simulink model "DBX_model_all"  (R2015a)
settings: Solver=ode2  SolverMode=SingleTasking  StartTime=0.0  StopTime=10  FixedStep=T_sim  RelTol=1e-3
undefined symbols (not defined in the file): A_M, Alpha_unique_rad, as, B_span, Beta_unique_rad, C_D_q, C_l, C_l_delta_a_Asim, C_l_delta_rv_Asim, C_l_p, C_l_r, C_Lift_q, C_m, C_m_q, C_n, C_n_delta_a_Asim, C_n_delta_rv_Asim, C_n_p, C_n_r, C_X, C_Y, C_Y_delta_rv_Asim, C_Y_p, C_Y_r, C_Z, CG, CMA, DBX_aero, DBX_aero_param, delta_elev_unique_rad, DOWN_0, EAST_0, F, g, h_1, h_2, h_3, I_BAC, Initial_Omegas, Initial_Torques, Ion, L_M, Lithium, m, MIL, NORTH_0, P_0, Q_0, R_0, Rotation_sign, Servo_calib, T_sim, U_0, V_0, W_0
libraries: simulink x19, DBX_model x14, aerolibwind2 x12, aerolibasang x9, aerolibadyn x4, aerolibatmos2 x2, powerlib x2, aerolibtransform2 x1, electricdrivelib x1
(part 2 of 3)

== system DBX_model_all/Aeromodel/Aero model V2 parametric/Wind Model ==
  note: Wind Models
  Alt (m) : Inport
  DCM : Inport  Port=2
  V_e (m/s) : Inport  Port=3
  Bias : Bias  Bias=eps
  Bias1 : Bias  Bias=eps
  Dot Product : DotProduct  SaturateOnIntegerOverflow=on  OutDataTypeStr=Inherit: Inherit via internal rule
  Dryden Wind Turbulence Model (Continuous (+q +r)) : aerolibwind2/Dryden Wind Turbulence Model  (Continuous (+q -r))  units=Metric (MKS)  spec=MIL-F-8785C  model=Continuous Von Karman (+q -r)  W20=0  Wdeg=90  TurbProb=2x10^-1  L_high=533.4  Wingspan=B_span  ts=0.2  Seed=[23341 23342 23343 23344]  T_on=on
  Horizontal Wind Model : aerolibwind2/Horizontal Wind Model  units=Metric (MKS)  Vw_source=Internal  Vwind=0  W_source=Internal  Wdeg=-60
  Sum : Sum  Inputs=+++  SaturateOnIntegerOverflow=on  InputSameDT=on  OutDataTypeStr=Inherit: Same as first input
  V : Math  Operator=sqrt  SaturateOnIntegerOverflow=on
  Wind Shear Model : aerolibwind2/Wind Shear Model  units=Metric (MKS)  phase=Category C - Terminal Flight Phase  W_20=0  Wdeg=0
  V_wind : Outport
  omega_wind : Outport  Port=2
  wires:
  Wind Shear Model/1 -> Sum/1
  Horizontal Wind Model/1 -> Sum/2
  Alt (m)/1 -> Dryden Wind Turbulence Model (Continuous (+q +r))/1, Wind Shear Model/1
  DCM/1 -> Horizontal Wind Model/1, Dryden Wind Turbulence Model (Continuous (+q +r))/3, Wind Shear Model/2
  Sum/1 -> Bias1/1
  Dryden Wind Turbulence Model (Continuous (+q +r))/2 -> omega_wind/1
  Dot Product/1 -> V/1
  V_e (m/s)/1 -> Dot Product/2, Dot Product/1
  Dryden Wind Turbulence Model (Continuous (+q +r))/1 -> Sum/3
  V/1 -> Bias/1
  Bias/1 -> Dryden Wind Turbulence Model (Continuous (+q +r))/2
  Bias1/1 -> V_wind/1

== system DBX_model_all/Aeromodel/Aero model aerosonde/Aerodynamics ==
  note: Aerodynamic Model
  note: Aerodynamic Coefficients
  note: Aerodynamic Parameters
  note: Outputs
  note: Inputs
  AeroCon : Inport  PortDimensions=[4 1]
  VelB : Inport  Port=2  PortDimensions=[3 1]
  Rates : Inport  Port=3  PortDimensions=[3 1]
  VelBdot : Inport  Port=4
  WindB : Inport  Port=5  PortDimensions=[3 1]
  WindRates : Inport  Port=6  PortDimensions=[3 1]
  rho : Inport  Port=7  PortDimensions=1
  "a " : Inport  Port=8  PortDimensions=1
  Force Coefficients : Subsystem
  Moment Coefficients : Subsystem
  Mux : Mux  Inputs=2
  Sum : Sum  Inputs=|+-  SaturateOnIntegerOverflow=on  InputSameDT=on  OutDataTypeStr=Inherit: Same as first input
  Wind-axes Velocities : Subsystem
  AeroCoeff_ba : Outport
  VelW : Outport  Port=2
  qbar (pdyn) : Outport  Port=3
  VBetaAlpha : Outport  Port=4
  wires:
  VelBdot/1 -> Wind-axes Velocities/5(VelBdot)
  Wind-axes Velocities/4(alphadot) -> Force Coefficients/3(AlphaDot), Moment Coefficients/3(AlphaDot)
  WindB/1 -> Wind-axes Velocities/2(WindB)
  Mux/1 -> AeroCoeff_ba/1
  Moment Coefficients/1("[-Cl, Cm, -Cn]") -> Mux/2
  Force Coefficients/1("[-CD, CY, -CL]") -> Mux/1
  rho/1 -> Wind-axes Velocities/4(rho)
  VelB/1 -> Wind-axes Velocities/1(VelB)
  "a "/1 -> Wind-axes Velocities/3(a)  "speed of sound"
  AeroCon/1 -> Moment Coefficients/2(Control), Force Coefficients/2(Control)
  Wind-axes Velocities/2(Mach) -> Moment Coefficients/5(Mach), Force Coefficients/5(Mach)
  Wind-axes Velocities/3(qbar (pdyn)) -> qbar (pdyn)/1
  Rates/1 -> Sum/1
  WindRates/1 -> Sum/2
  Sum/1 -> Moment Coefficients/4(AngularRates), Force Coefficients/4(AngularRates)  "pqr"
  Wind-axes Velocities/1(VBetaAlpha) -> VBetaAlpha/1, Moment Coefficients/1(VBetaAlpha), VelW/1, Force Coefficients/1(VBetaAlpha)

== system DBX_model_all/Aeromodel/Aero model aerosonde/Deflex mixer ==
  note: Control inputs:
      |
      |
      | 7. Rudervator Left (rad)
      | 8. Rudervator Right (rad)
      | 9. Aileron Left (rad)
      | 10. Aielron Right (rad)
  Sups_control : Inport
  Add : Sum  Inputs=|+-
  Add1 : Sum  Inputs=|++
  Add2 : Sum  Inputs=|+-
  Demux : Demux
  Gain : Gain  Gain=1/2
  Gain1 : Gain  Gain=1/2
  Gain2 : Gain  Gain=1/2
  delta_ail_Asim : Outport
  delta_rv_sim : Outport  Port=2
  delta_rv_Asim : Outport  Port=3
  wires:
  Sups_control/1 -> Demux/1
  Demux/3 -> Add/1
  Demux/4 -> Add/2
  Add/1 -> Gain/1
  Gain/1 -> delta_ail_Asim/1
  Demux/1 -> Add2/1, Add1/1
  Demux/2 -> Add2/2, Add1/2
  Add2/1 -> Gain1/1
  Add1/1 -> Gain2/1
  Gain2/1 -> delta_rv_sim/1
  Gain1/1 -> delta_rv_Asim/1

== system DBX_model_all/Aeromodel/Aero model aerosonde/Wind Model ==
  note: Wind Models
  Alt (m) : Inport
  DCM : Inport  Port=2
  V_e (m/s) : Inport  Port=3
  Dot Product : DotProduct  SaturateOnIntegerOverflow=on  OutDataTypeStr=Inherit: Inherit via internal rule
  Dryden Wind Turbulence Model (Continuous (+q +r)) : aerolibwind2/Dryden Wind Turbulence Model  (Continuous (+q -r))  units=Metric (MKS)  spec=MIL-F-8785C  model=Continuous Von Karman (+q -r)  W20=0  Wdeg=90  TurbProb=2x10^-1  L_high=533.4  Wingspan=B_span  ts=0.02  Seed=[23341 23342 23343 23344]  T_on=on
  Horizontal Wind Model : aerolibwind2/Horizontal Wind Model  units=Metric (MKS)  Vw_source=Internal  Vwind=0  W_source=Internal  Wdeg=-60
  Sum : Sum  Inputs=+++  SaturateOnIntegerOverflow=on  InputSameDT=on  OutDataTypeStr=Inherit: Same as first input
  V : Math  Operator=sqrt  SaturateOnIntegerOverflow=on
  Wind Shear Model : aerolibwind2/Wind Shear Model  units=Metric (MKS)  phase=Category C - Terminal Flight Phase  W_20=0  Wdeg=0
  V_wind : Outport
  omega_wind : Outport  Port=2
  wires:
  V/1 -> Dryden Wind Turbulence Model (Continuous (+q +r))/2
  Dryden Wind Turbulence Model (Continuous (+q +r))/1 -> Sum/3
  V_e (m/s)/1 -> Dot Product/2, Dot Product/1
  Dot Product/1 -> V/1
  Dryden Wind Turbulence Model (Continuous (+q +r))/2 -> omega_wind/1
  Sum/1 -> V_wind/1
  DCM/1 -> Horizontal Wind Model/1, Dryden Wind Turbulence Model (Continuous (+q +r))/3, Wind Shear Model/2
  Alt (m)/1 -> Dryden Wind Turbulence Model (Continuous (+q +r))/1, Wind Shear Model/1
  Horizontal Wind Model/1 -> Sum/2
  Wind Shear Model/1 -> Sum/1

== system DBX_model_all/Aeromodel/Aero model V1/Aerodynamics/Deflex mixer ==
  note: Control inputs:
      |
      |
      | 7. Rudervator Left (rad)
      | 8. Rudervator Right (rad)
      | 9. Aileron Left (rad)
      | 10. Aielron Right (rad)
  Sups_control : Inport
  Add : Sum  Inputs=|+-
  Add1 : Sum  Inputs=|++
  Add2 : Sum  Inputs=|+-
  Demux : Demux
  Gain : Gain  Gain=1/2
  Gain1 : Gain  Gain=1/2
  Gain2 : Gain  Gain=1/2
  delta_ail_Asim : Outport
  delta_rv_sim : Outport  Port=2
  delta_rv_Asim : Outport  Port=3
  wires:
  Sups_control/1 -> Demux/1
  Demux/3 -> Add/1
  Demux/4 -> Add/2
  Add/1 -> Gain/1
  Gain/1 -> delta_ail_Asim/1
  Demux/1 -> Add2/1, Add1/1
  Demux/2 -> Add2/2, Add1/2
  Add2/1 -> Gain1/1
  Add1/1 -> Gain2/1
  Gain2/1 -> delta_rv_sim/1
  Gain1/1 -> delta_rv_Asim/1

== system DBX_model_all/Aeromodel/Aero model V1/Aerodynamics/Force Coefficients ==
  note: Con Cariño para Luis :P
  note: Deflexiones efectivas:
      |
      | delta_ail_Asim
      | delta_rv_sim
      | delta_rv_Asim
  alpha : Inport
  beta : Inport  Port=2
  body_rates_adim : Inport  Port=3
  defl_control : Inport  Port=4
  C_X_T : Subsystem
  C_Y_T : Subsystem
  C_Z_T : Subsystem
  Mux : Mux  Inputs=3
  "[C_X_T, C_Y_T, C_Z_T]" : Outport
  wires:
  alpha/1 -> C_Z_T/1(alpha), C_Y_T/1(alpha), C_X_T/1(alpha)
  beta/1 -> C_Z_T/2(beta), C_Y_T/2(beta), C_X_T/2(beta)
  body_rates_adim/1 -> C_Z_T/3(body_rates_adim), C_Y_T/3(body_rates_adim), C_X_T/3(body_rates_adim)
  defl_control/1 -> C_Z_T/4(defl_control), C_Y_T/4(defl_control), C_X_T/4(defl_control)
  C_Y_T/1(C_Y_T) -> Mux/2
  Mux/1 -> "[C_X_T, C_Y_T, C_Z_T]"/1
  C_X_T/1(C_X_T) -> Mux/1
  C_Z_T/1(C_Z_T) -> Mux/3

== system DBX_model_all/Aeromodel/Aero model V1/Aerodynamics/Moment Coefficients ==
  note: Con Cariño para Luis :P
  note: Deflexiones efectivas:
      |
      | delta_ail_Asim
      | delta_rv_sim
      | delta_rv_Asim
  alpha : Inport
  beta : Inport  Port=2
  body_rates_adim : Inport  Port=3  PortDimensions=[3 1]
  defl_control : Inport  Port=4
  C_l_T : Subsystem
  C_m_T : Subsystem
  C_n_T : Subsystem
  Mux : Mux  Inputs=3
  "[C_l_T, C_m_T, C_n_T]" : Outport
  wires:
  alpha/1 -> C_n_T/1(alpha), C_m_T/1(alpha), C_l_T/1(alpha)
  beta/1 -> C_n_T/2(beta), C_m_T/2(beta), C_l_T/2(beta)
  body_rates_adim/1 -> C_n_T/3(body_rates_adim), C_m_T/3(body_rates_adim), C_l_T/3(body_rates_adim)
  defl_control/1 -> C_n_T/4(defl_control), C_m_T/4(defl_control), C_l_T/4(defl_control)
  Mux/1 -> "[C_l_T, C_m_T, C_n_T]"/1
  C_l_T/1(C_l_T) -> Mux/1
  C_m_T/1(C_m_T) -> Mux/2
  C_n_T/1(C_n_T) -> Mux/3

== system DBX_model_all/Aeromodel/Aero model V1/Aerodynamics/Wind-axes Velocities ==
  Vb : Inport
  V_wind_b : Inport  Port=2
  a : Inport  Port=3
  rho : Inport  Port=4
  Vb_dot : Inport  Port=5
  Calculate alphadot : Subsystem
  Derivative : Derivative  CoefficientInTFapproximation=500
  Dynamic Pressure : aerolibasang/Dynamic Pressure
  "Incidence, Sideslip, & Airspeed" : aerolibasang/Incidence, Sideslip, & Airspeed
  Sum1 : Sum  Inputs=|+-  SaturateOnIntegerOverflow=on  InputSameDT=on  OutDataTypeStr=Inherit: Same as first input
  Sum2 : Sum  Inputs=-+|  SaturateOnIntegerOverflow=on  InputSameDT=on  OutDataTypeStr=Inherit: Same as first input
  Terminator : Terminator
  qbar (pdyn) : Outport
  alphadot : Outport  Port=2
  alpha : Outport  Port=3
  beta : Outport  Port=4
  TAS : Outport  Port=5
  wires:
  Derivative/1 -> Sum2/1
  Sum2/1 -> Calculate alphadot/1("[Udot Vdot Wdot]")
  Vb_dot/1 -> Sum2/2
  Calculate alphadot/1(alphadot) -> alphadot/1
  Dynamic Pressure/1 -> qbar (pdyn)/1
  rho/1 -> Dynamic Pressure/2
  V_wind_b/1 -> Derivative/1, Sum1/2
  Vb/1 -> Sum1/1
  Sum1/1 -> Calculate alphadot/2("[U V W]"), Dynamic Pressure/1, "Incidence, Sideslip, & Airspeed"/1
  "Incidence, Sideslip, & Airspeed"/3 -> TAS/1
  "Incidence, Sideslip, & Airspeed"/2 -> beta/1
  "Incidence, Sideslip, & Airspeed"/1 -> alpha/1
  a/1 -> Terminator/1

== system DBX_model_all/Aeromodel/Aero model V2/Aerodynamics/Deflex mixer ==
  note: Control inputs:
      |
      |
      | 7. Rudervator Left (rad)
      | 8. Rudervator Right (rad)
      | 9. Aileron Left (rad)
      | 10. Aielron Right (rad)
  Sups_control : Inport
  Add : Sum  Inputs=|+-
  Add1 : Sum  Inputs=|++
  Add2 : Sum  Inputs=|+-
  Demux : Demux
  Gain : Gain  Gain=1/2
  Gain1 : Gain  Gain=1/2
  Gain2 : Gain  Gain=1/2
  delta_ail_Asim : Outport
  delta_rv_sim : Outport  Port=2
  delta_rv_Asim : Outport  Port=3
  wires:
  Gain1/1 -> delta_rv_Asim/1
  Gain2/1 -> delta_rv_sim/1
  Add1/1 -> Gain2/1
  Add2/1 -> Gain1/1
  Demux/2 -> Add1/2, Add2/2
  Demux/1 -> Add1/1, Add2/1
  Gain/1 -> delta_ail_Asim/1
  Add/1 -> Gain/1
  Demux/4 -> Add/2
  Demux/3 -> Add/1
  Sups_control/1 -> Demux/1

== system DBX_model_all/Aeromodel/Aero model V2/Aerodynamics/Force Coefficients ==
  note: Con Cariño para Luis :P
  note: Deflexiones del modelo Aero:
      |
      | delta_ail
      | delta_elev
      | delta_rudder
  alpha : Inport
  beta : Inport  Port=2
  body_rates_adim : Inport  Port=3
  defl_control : Inport  Port=4
  C_X_T : Subsystem
  C_Y_T : Subsystem
  C_Z_T : Subsystem
  Mux : Mux  Inputs=3
  "[C_X_T, C_Y_T, C_Z_T]" : Outport
  wires:
  C_Z_T/1(C_Z_T) -> Mux/3
  C_X_T/1(C_X_T) -> Mux/1
  Mux/1 -> "[C_X_T, C_Y_T, C_Z_T]"/1
  C_Y_T/1(C_Y_T) -> Mux/2
  defl_control/1 -> C_X_T/4(defl_control), C_Z_T/4(defl_control), C_Y_T/4(defl_control)
  body_rates_adim/1 -> C_X_T/3(body_rates_adim), C_Z_T/3(body_rates_adim), C_Y_T/3(body_rates_adim)
  beta/1 -> C_X_T/2(beta), C_Z_T/2(beta), C_Y_T/2(beta)
  alpha/1 -> C_X_T/1(alpha), C_Z_T/1(alpha), C_Y_T/1(alpha)

== system DBX_model_all/Aeromodel/Aero model V2/Aerodynamics/Moment Coefficients ==
  note: Con Cariño para Luis :P
  note: Deflexiones del modelo Aero:
      |
      | delta_ail
      | delta_elev
      | delta_rudder
  alpha : Inport
  beta : Inport  Port=2
  body_rates_adim : Inport  Port=3  PortDimensions=[3 1]
  defl_control : Inport  Port=4
  C_l_T : Subsystem
  C_m_T : Subsystem
  C_n_T : Subsystem
  Mux : Mux  Inputs=3
  "[C_l_T, C_m_T, C_n_T]" : Outport
  wires:
  C_n_T/1(C_n_T) -> Mux/3
  C_m_T/1(C_m_T) -> Mux/2
  C_l_T/1(C_l_T) -> Mux/1
  Mux/1 -> "[C_l_T, C_m_T, C_n_T]"/1
  defl_control/1 -> C_l_T/4(defl_control), C_n_T/4(defl_control), C_m_T/4(defl_control)
  body_rates_adim/1 -> C_l_T/3(body_rates_adim), C_n_T/3(body_rates_adim), C_m_T/3(body_rates_adim)
  beta/1 -> C_l_T/2(beta), C_n_T/2(beta), C_m_T/2(beta)
  alpha/1 -> C_l_T/1(alpha), C_n_T/1(alpha), C_m_T/1(alpha)

== system DBX_model_all/Aeromodel/Aero model V2/Aerodynamics/Wind-axes Velocities ==
  Vb : Inport
  V_wind_b : Inport  Port=2
  a : Inport  Port=3
  rho : Inport  Port=4
  Vb_dot : Inport  Port=5
  Calculate alphadot : Subsystem
  Derivative : Derivative  CoefficientInTFapproximation=500
  Dynamic Pressure : aerolibasang/Dynamic Pressure
  "Incidence, Sideslip, & Airspeed" : aerolibasang/Incidence, Sideslip, & Airspeed
  Sum1 : Sum  Inputs=|+-  SaturateOnIntegerOverflow=on  InputSameDT=on  OutDataTypeStr=Inherit: Same as first input
  Sum2 : Sum  Inputs=-+|  SaturateOnIntegerOverflow=on  InputSameDT=on  OutDataTypeStr=Inherit: Same as first input
  Terminator : Terminator
  qbar (pdyn) : Outport
  alphadot : Outport  Port=2
  alpha : Outport  Port=3
  beta : Outport  Port=4
  TAS : Outport  Port=5
  wires:
  a/1 -> Terminator/1
  "Incidence, Sideslip, & Airspeed"/1 -> alpha/1
  "Incidence, Sideslip, & Airspeed"/2 -> beta/1
  "Incidence, Sideslip, & Airspeed"/3 -> TAS/1
  Sum1/1 -> "Incidence, Sideslip, & Airspeed"/1, Dynamic Pressure/1, Calculate alphadot/2("[U V W]")
  Vb/1 -> Sum1/1
  V_wind_b/1 -> Sum1/2, Derivative/1
  rho/1 -> Dynamic Pressure/2
  Dynamic Pressure/1 -> qbar (pdyn)/1
  Calculate alphadot/1(alphadot) -> alphadot/1
  Vb_dot/1 -> Sum2/2
  Sum2/1 -> Calculate alphadot/1("[Udot Vdot Wdot]")
  Derivative/1 -> Sum2/1

== system DBX_model_all/Aeromodel/Aero model V2 parametric/Aerodynamics/Deflex mixer ==
  note: Control inputs:
      |
      |
      | 7. Rudervator Left (rad)
      | 8. Rudervator Right (rad)
      | 9. Aileron Left (rad)
      | 10. Aielron Right (rad)
  Sups_control : Inport
  Add : Sum  Inputs=|+-
  Add1 : Sum  Inputs=|++
  Add2 : Sum  Inputs=|+-
  Demux : Demux
  Gain : Gain  Gain=1/2
  Gain1 : Gain  Gain=1/2
  Gain2 : Gain  Gain=1/2
  delta_ail_Asim : Outport
  delta_rv_sim : Outport  Port=2
  delta_rv_Asim : Outport  Port=3
  wires:
  Gain1/1 -> delta_rv_Asim/1
  Gain2/1 -> delta_rv_sim/1
  Add1/1 -> Gain2/1
  Add2/1 -> Gain1/1
  Demux/2 -> Add1/2, Add2/2
  Demux/1 -> Add1/1, Add2/1
  Gain/1 -> delta_ail_Asim/1
  Add/1 -> Gain/1
  Demux/4 -> Add/2
  Demux/3 -> Add/1
  Sups_control/1 -> Demux/1

== system DBX_model_all/Aeromodel/Aero model V2 parametric/Aerodynamics/Force Coefficients ==
  note: Con Cariño para Luis :P
  note: Deflexiones del modelo Aero:
      |
      | delta_ail
      | delta_elev
      | delta_rudder
  alpha : Inport
  beta : Inport  Port=2
  body_rates_adim : Inport  Port=3
  defl_control : Inport  Port=4
  C_X_T : Subsystem
  C_Y_T : Subsystem
  C_Z_T : Subsystem
  Mux : Mux  Inputs=3
  "[C_X_T, C_Y_T, C_Z_T]" : Outport
  wires:
  C_Z_T/1(C_Z_T) -> Mux/3
  C_X_T/1(C_X_T) -> Mux/1
  Mux/1 -> "[C_X_T, C_Y_T, C_Z_T]"/1
  C_Y_T/1(C_Y_T) -> Mux/2
  defl_control/1 -> C_X_T/4(defl_control), C_Z_T/4(defl_control), C_Y_T/4(defl_control)
  body_rates_adim/1 -> C_X_T/3(body_rates_adim), C_Z_T/3(body_rates_adim), C_Y_T/3(body_rates_adim)
  beta/1 -> C_X_T/2(beta), C_Z_T/2(beta), C_Y_T/2(beta)
  alpha/1 -> C_X_T/1(alpha), C_Z_T/1(alpha), C_Y_T/1(alpha)

== system DBX_model_all/Aeromodel/Aero model V2 parametric/Aerodynamics/Moment Coefficients ==
  note: Con Cariño para Luis :P
  note: Deflexiones del modelo Aero:
      |
      | delta_ail
      | delta_elev
      | delta_rudder
  alpha : Inport
  beta : Inport  Port=2
  body_rates_adim : Inport  Port=3  PortDimensions=[3 1]
  defl_control : Inport  Port=4
  C_l_T : Subsystem
  C_m_T : Subsystem
  C_n_T : Subsystem
  Mux : Mux  Inputs=3
  "[C_l_T, C_m_T, C_n_T]" : Outport
  wires:
  C_n_T/1(C_n_T) -> Mux/3
  C_m_T/1(C_m_T) -> Mux/2
  C_l_T/1(C_l_T) -> Mux/1
  Mux/1 -> "[C_l_T, C_m_T, C_n_T]"/1
  defl_control/1 -> C_l_T/4(defl_control), C_n_T/4(defl_control), C_m_T/4(defl_control)
  body_rates_adim/1 -> C_l_T/3(body_rates_adim), C_n_T/3(body_rates_adim), C_m_T/3(body_rates_adim)
  beta/1 -> C_l_T/2(beta), C_n_T/2(beta), C_m_T/2(beta)
  alpha/1 -> C_l_T/1(alpha), C_n_T/1(alpha), C_m_T/1(alpha)

== system DBX_model_all/Aeromodel/Aero model V2 parametric/Aerodynamics/Wind-axes Velocities ==
  Vb : Inport
  V_wind_b : Inport  Port=2
  a : Inport  Port=3
  rho : Inport  Port=4
  Vb_dot : Inport  Port=5
  Calculate alphadot : Subsystem
  Derivative : Derivative  CoefficientInTFapproximation=500
  Dynamic Pressure : aerolibasang/Dynamic Pressure
  "Incidence, Sideslip, & Airspeed" : aerolibasang/Incidence, Sideslip, & Airspeed
  Sum1 : Sum  Inputs=|+-  SaturateOnIntegerOverflow=on  InputSameDT=on  OutDataTypeStr=Inherit: Same as first input
  Sum2 : Sum  Inputs=-+|  SaturateOnIntegerOverflow=on  InputSameDT=on  OutDataTypeStr=Inherit: Same as first input
  Terminator : Terminator
  qbar (pdyn) : Outport
  alphadot : Outport  Port=2
  alpha : Outport  Port=3
  beta : Outport  Port=4
  TAS : Outport  Port=5
  wires:
  a/1 -> Terminator/1
  "Incidence, Sideslip, & Airspeed"/1 -> alpha/1
  "Incidence, Sideslip, & Airspeed"/2 -> beta/1
  "Incidence, Sideslip, & Airspeed"/3 -> TAS/1
  Sum1/1 -> "Incidence, Sideslip, & Airspeed"/1, Dynamic Pressure/1, Calculate alphadot/2("[U V W]")
  Vb/1 -> Sum1/1
  V_wind_b/1 -> Sum1/2, Derivative/1
  rho/1 -> Dynamic Pressure/2
  Dynamic Pressure/1 -> qbar (pdyn)/1
  Calculate alphadot/1(alphadot) -> alphadot/1
  Vb_dot/1 -> Sum2/2
  Sum2/1 -> Calculate alphadot/1("[Udot Vdot Wdot]")
  Derivative/1 -> Sum2/1

== system DBX_model_all/Aeromodel/Aero model aerosonde/Aerodynamics/Force Coefficients ==
  note: Force coefficients
  VBetaAlpha : Inport  PortDimensions=[3 1]
  Control : Inport  Port=2  PortDimensions=[4 1]
  AlphaDot : Inport  Port=3
  AngularRates : Inport  Port=4  PortDimensions=[3 1]
  Mach : Inport  Port=5  PortDimensions=1
  2c : Gain  Gain=2  SaturateOnIntegerOverflow=on  OutDataTypeStr=Inherit: Same as input  ParamDataTypeStr=Inherit: Same as input
  ChSign : Gain  Gain=-1  SaturateOnIntegerOverflow=on  OutDataTypeStr=Inherit: Same as input  ParamDataTypeStr=Inherit: Same as input
  ChSign1 : Gain  Gain=-1  SaturateOnIntegerOverflow=on  OutDataTypeStr=Inherit: Same as input  ParamDataTypeStr=Inherit: Same as input
  DCM' : Math  Operator=transpose  SaturateOnIntegerOverflow=on
  Demux2 : Demux  Outputs=3
  Direction Cosine Matrix Body to Wind : aerolibtransform2/Direction Cosine Matrix Body to Wind
  Drag Coefficients : Subsystem
  Lift Coefficients : Subsystem
  Mux : Mux  Inputs=3
  Mux1 : Mux  Inputs=2
  Side Force Coefficients : Subsystem
  transform to body axes : Product  Inputs=**  Multiplication=Matrix(*)  SaturateOnIntegerOverflow=on  InputSameDT=on  OutDataTypeStr=Inherit: Same as first input
  "[-CD, CY, -CL]" : Outport
  wires:
  Mux1/1 -> Direction Cosine Matrix Body to Wind/1
  DCM'/1 -> transform to body axes/1
  Mux/1 -> transform to body axes/2
  Direction Cosine Matrix Body to Wind/1 -> DCM'/1
  transform to body axes/1 -> "[-CD, CY, -CL]"/1
  Demux2/2 -> Mux1/2, Side Force Coefficients/1(beta)
  Demux2/1 -> 2c/1
  VBetaAlpha/1 -> Demux2/1
  ChSign1/1 -> Mux/3
  ChSign/1 -> Mux/1
  Side Force Coefficients/1(CY) -> Mux/2
  Drag Coefficients/1(CD) -> ChSign/1
  Lift Coefficients/1(CL) -> Drag Coefficients/3(CL), ChSign1/1
  Mach/1 -> Drag Coefficients/2(Mach), Lift Coefficients/6(Mach)
  AngularRates/1 -> Side Force Coefficients/3(angular rates), Lift Coefficients/4(pqr)
  AlphaDot/1 -> Lift Coefficients/3(alphadot)
  Control/1 -> Side Force Coefficients/2(control), Lift Coefficients/2(control), Drag Coefficients/1(control)
  Demux2/3 -> Lift Coefficients/1(alpha), Mux1/1
  2c/1 -> Side Force Coefficients/4(2V_a), Lift Coefficients/5(2V_a)

== system DBX_model_all/Aeromodel/Aero model aerosonde/Aerodynamics/Moment Coefficients ==
  note: Moment coefficients
  VBetaAlpha : Inport  PortDimensions=[3 1]
  Control : Inport  Port=2  PortDimensions=[4 1]
  AlphaDot : Inport  Port=3
  AngularRates : Inport  Port=4  PortDimensions=[3 1]
  Mach : Inport  Port=5  PortDimensions=1
  2c : Gain  Gain=2  SaturateOnIntegerOverflow=on  OutDataTypeStr=Inherit: Same as input  ParamDataTypeStr=Inherit: Same as input
  Demux1 : Demux  Outputs=3
  Mux : Mux  Inputs=3
  Pitch Moment Coefficients : Subsystem
  Roll Moment Coefficients : Subsystem
  Yaw Moment Coefficients : Subsystem
  "[-Cl, Cm, -Cn]" : Outport
  wires:
  Demux1/2 -> Yaw Moment Coefficients/1(beta), Roll Moment Coefficients/1(beta)
  Demux1/3 -> Pitch Moment Coefficients/1(alpha)
  Mach/1 -> Pitch Moment Coefficients/6(Mach)
  Yaw Moment Coefficients/1(Cn) -> Mux/3
  VBetaAlpha/1 -> Demux1/1
  2c/1 -> Pitch Moment Coefficients/5(2V_a), Yaw Moment Coefficients/4(2V_a), Roll Moment Coefficients/4(2V)
  Demux1/1 -> 2c/1
  Control/1 -> Yaw Moment Coefficients/2(control), Pitch Moment Coefficients/2(control), Roll Moment Coefficients/2(control)
  AlphaDot/1 -> Pitch Moment Coefficients/3(alphadot)
  AngularRates/1 -> Roll Moment Coefficients/3(angular rates), Yaw Moment Coefficients/3(angular rates), Pitch Moment Coefficients/4(pqr)
  Mux/1 -> "[-Cl, Cm, -Cn]"/1
  Pitch Moment Coefficients/1(Cm) -> Mux/2
  Roll Moment Coefficients/1(Cl) -> Mux/1

== system DBX_model_all/Aeromodel/Aero model aerosonde/Aerodynamics/Wind-axes Velocities ==
  VelB : Inport
  WindB : Inport  Port=2
  a : Inport  Port=3
  rho : Inport  Port=4
  VelBdot : Inport  Port=5
  Calculate alphadot : Subsystem
  Derivative : Derivative
  Dynamic Pressure : aerolibasang/Dynamic Pressure
  "Incidence, Sideslip, & Airspeed" : aerolibasang/Incidence, Sideslip, & Airspeed
  Mach Number : aerolibasang/Mach Number
  Mux1 : Mux  Inputs=3
  Sum1 : Sum  Inputs=|+-  SaturateOnIntegerOverflow=on  InputSameDT=on  OutDataTypeStr=Inherit: Same as first input
  Sum2 : Sum  Inputs=-+|  SaturateOnIntegerOverflow=on  InputSameDT=on  OutDataTypeStr=Inherit: Same as first input
  VBetaAlpha : Outport
  Mach : Outport  Port=2
  qbar (pdyn) : Outport  Port=3
  alphadot : Outport  Port=4
  wires:
  Derivative/1 -> Sum2/1
  Sum2/1 -> Calculate alphadot/1("[Udot Vdot Wdot]")
  VelBdot/1 -> Sum2/2
  Calculate alphadot/1(alphadot) -> alphadot/1
  "Incidence, Sideslip, & Airspeed"/2 -> Mux1/2
  "Incidence, Sideslip, & Airspeed"/1 -> Mux1/3
  Dynamic Pressure/1 -> qbar (pdyn)/1
  rho/1 -> Dynamic Pressure/2
  a/1 -> Mach Number/2
  Mach Number/1 -> Mach/1
  WindB/1 -> Derivative/1, Sum1/2
  VelB/1 -> Sum1/1
  Mux1/1 -> VBetaAlpha/1
  "Incidence, Sideslip, & Airspeed"/3 -> Mux1/1
  Sum1/1 -> Calculate alphadot/2("[U V W]"), Dynamic Pressure/1, Mach Number/1, "Incidence, Sideslip, & Airspeed"/1

== system DBX_model_all/Aeromodel/Aero model V1/Aerodynamics/Force Coefficients/C_X_T ==
  note: Deflexiones efectivas:
      |
      | delta_ail_Asim
      | delta_rv_sim
      | delta_rv_Asim
  alpha : Inport
  beta : Inport  Port=2
  body_rates_adim : Inport  Port=3  PortDimensions=[3 1]
  defl_control : Inport  Port=4
  Add : Sum  Inputs=++|
  Add1 : Sum  Inputs=-+|
  C_D_q : Constant  Value=C_D_q
  C_Lift_q : Constant  Value=C_Lift_q
  C_X : Lookup_n-D  NumberOfTableDimensions=3  BreakpointsForDimension1=Alpha_unique_rad  BreakpointsForDimension2=Beta_unique_rad  BreakpointsForDimension3=delta_elev_unique_rad  Table=C_X  DiagnosticForOutOfRangeInput=Warning  RemoveProtectionInput=on  InternalRulePriority=Speed  RndMeth=Simplest  InputSameDT=on
  Divide : Product  Inputs=**
  Divide1 : Product  Inputs=**
  Divide2 : Product  Inputs=**
  Selector : Selector  InputPortWidth=3  Indices=2
  Selector1 : Selector  InputPortWidth=3  Indices=2
  cos : Trigonometry  Operator=cos
  sin : Trigonometry
  C_X_T : Outport
  wires:
  alpha/1 -> cos/1, sin/1, C_X/1
  beta/1 -> C_X/2
  body_rates_adim/1 -> Selector/1
  Selector/1 -> Divide/1
  C_X/1 -> Add/1
  Divide/1 -> Add/2
  Add/1 -> C_X_T/1
  defl_control/1 -> Selector1/1
  Selector1/1 -> C_X/3
  sin/1 -> Divide1/1
  C_Lift_q/1 -> Divide1/2
  cos/1 -> Divide2/1
  C_D_q/1 -> Divide2/2
  Divide1/1 -> Add1/2
  Divide2/1 -> Add1/1
  Add1/1 -> Divide/2

== system DBX_model_all/Aeromodel/Aero model V1/Aerodynamics/Force Coefficients/C_Y_T ==
  note: Deflexiones efectivas:
      |
      | delta_ail_Asim
      | delta_rv_sim
      | delta_rv_Asim
  alpha : Inport
  beta : Inport  Port=2
  body_rates_adim : Inport  Port=3  PortDimensions=[3 1]
  defl_control : Inport  Port=4
  Add : Sum  Inputs=++++
  C_Y : Lookup_n-D  BreakpointsForDimension1=Alpha_unique_rad  BreakpointsForDimension2=Beta_unique_rad  Table=C_Y  DiagnosticForOutOfRangeInput=Warning  RemoveProtectionInput=on  InternalRulePriority=Speed  RndMeth=Simplest  InputSameDT=on
  C_Y_delta_rv : Constant  Value=C_Y_delta_rv_Asim
  C_Y_p : Constant  Value=C_Y_p
  C_Y_r : Constant  Value=C_Y_r
  Divide : Product  Inputs=**
  Divide1 : Product  Inputs=**
  Divide2 : Product  Inputs=**
  Selector : Selector  InputPortWidth=3  Indices=3
  Selector1 : Selector  InputPortWidth=3
  Selector2 : Selector  InputPortWidth=3  Indices=3
  C_Y_T : Outport
  wires:
  alpha/1 -> C_Y/1
  beta/1 -> C_Y/2
  Selector/1 -> Divide/1
  C_Y_r/1 -> Divide/2
  body_rates_adim/1 -> Selector1/1, Selector/1
  Selector1/1 -> Divide1/1
  C_Y_p/1 -> Divide1/2
  defl_control/1 -> Selector2/1
  C_Y_delta_rv/1 -> Divide2/2
  Selector2/1 -> Divide2/1
  Divide2/1 -> Add/4
  Divide1/1 -> Add/3
  Divide/1 -> Add/2
  C_Y/1 -> Add/1
  Add/1 -> C_Y_T/1

== system DBX_model_all/Aeromodel/Aero model V1/Aerodynamics/Force Coefficients/C_Z_T ==
  note: Deflexiones efectivas:
      |
      | delta_ail_Asim
      | delta_rv_sim
      | delta_rv_Asim
  alpha : Inport
  beta : Inport  Port=2
  body_rates_adim : Inport  Port=3  PortDimensions=[3 1]
  defl_control : Inport  Port=4
  Add : Sum  Inputs=++|
  Add1 : Sum  Inputs=--|
  C_D_q : Constant  Value=C_D_q
  C_Lift_q : Constant  Value=C_Lift_q
  C_Z : Lookup_n-D  NumberOfTableDimensions=3  BreakpointsForDimension1=Alpha_unique_rad  BreakpointsForDimension2=Beta_unique_rad  BreakpointsForDimension3=delta_elev_unique_rad  Table=C_Z  DiagnosticForOutOfRangeInput=Warning  RemoveProtectionInput=on  InternalRulePriority=Speed  RndMeth=Simplest  InputSameDT=on
  Divide : Product  Inputs=**
  Divide1 : Product  Inputs=**
  Divide2 : Product  Inputs=**
  Selector : Selector  InputPortWidth=3  Indices=2
  Selector1 : Selector  InputPortWidth=3  Indices=2
  cos : Trigonometry  Operator=cos
  sin : Trigonometry
  C_Z_T : Outport
  wires:
  Add/1 -> C_Z_T/1
  Divide/1 -> Add/2
  C_Z/1 -> Add/1
  Selector/1 -> Divide/1
  body_rates_adim/1 -> Selector/1
  beta/1 -> C_Z/2
  alpha/1 -> cos/1, sin/1, C_Z/1
  defl_control/1 -> Selector1/1
  Selector1/1 -> C_Z/3
  cos/1 -> Divide1/1
  C_Lift_q/1 -> Divide1/2
  C_D_q/1 -> Divide2/2
  Divide1/1 -> Add1/2
  Divide2/1 -> Add1/1
  sin/1 -> Divide2/1
  Add1/1 -> Divide/2

== system DBX_model_all/Aeromodel/Aero model V1/Aerodynamics/Moment Coefficients/C_l_T ==
  note: Deflexiones efectivas:
      |
      | delta_ail_Asim
      | delta_rv_sim
      | delta_rv_Asim
  alpha : Inport
  beta : Inport  Port=2
  body_rates_adim : Inport  Port=3  PortDimensions=[3 1]
  defl_control : Inport  Port=4
  Add : Sum  Inputs=+++++
  C_l : Lookup_n-D  BreakpointsForDimension1=Alpha_unique_rad  BreakpointsForDimension2=Beta_unique_rad  Table=C_l  DiagnosticForOutOfRangeInput=Warning  RemoveProtectionInput=on  InternalRulePriority=Speed  RndMeth=Simplest  InputSameDT=on
  C_l_delta_a : Constant  Value=C_l_delta_a_Asim
  C_l_delta_rv : Constant  Value=C_l_delta_rv_Asim
  C_l_p : Constant  Value=C_l_p
  C_l_r : Constant  Value=C_l_r
  Divide{,1..3} (4 alike) : Product  Inputs=**
  Selector : Selector  InputPortWidth=3  Indices=3
  Selector1 : Selector  InputPortWidth=3  Indices=3
  Selector2 : Selector  InputPortWidth=3
  Selector3 : Selector  InputPortWidth=3
  C_l_T : Outport
  wires:
  alpha/1 -> C_l/1
  beta/1 -> C_l/2
  Add/1 -> C_l_T/1
  defl_control/1 -> Selector1/1, Selector2/1
  C_l_delta_a/1 -> Divide2/2
  Selector2/1 -> Divide2/1
  C_l_delta_rv/1 -> Divide1/2
  Selector1/1 -> Divide1/1
  C_l_r/1 -> Divide/2
  body_rates_adim/1 -> Selector3/1, Selector/1
  Selector3/1 -> Divide3/1
  C_l_p/1 -> Divide3/2
  Selector/1 -> Divide/1
  C_l/1 -> Add/1
  Divide/1 -> Add/2
  Divide3/1 -> Add/3
  Divide2/1 -> Add/4
  Divide1/1 -> Add/5

== system DBX_model_all/Aeromodel/Aero model V1/Aerodynamics/Moment Coefficients/C_m_T ==
  note: Deflexiones efectivas:
      |
      | delta_ail_Asim
      | delta_rv_sim
      | delta_rv_Asim
  alpha : Inport
  beta : Inport  Port=2
  body_rates_adim : Inport  Port=3  PortDimensions=[3 1]
  defl_control : Inport  Port=4
  Add : Sum  Inputs=++|
  C_m : Lookup_n-D  NumberOfTableDimensions=3  BreakpointsForDimension1=Alpha_unique_rad  BreakpointsForDimension2=Beta_unique_rad  BreakpointsForDimension3=delta_elev_unique_rad  Table=C_m  DiagnosticForOutOfRangeInput=Warning  RemoveProtectionInput=on  InternalRulePriority=Speed  RndMeth=Simplest  InputSameDT=on
  C_m_q : Constant  Value=C_m_q
  Divide : Product  Inputs=**
  Selector : Selector  InputPortWidth=3  Indices=2
  Selector2 : Selector  InputPortWidth=3  Indices=2
  C_m_T : Outport
  wires:
  alpha/1 -> C_m/1
  Selector/1 -> Divide/1
  C_m_q/1 -> Divide/2
  body_rates_adim/1 -> Selector/1
  defl_control/1 -> Selector2/1
  Divide/1 -> Add/2
  C_m/1 -> Add/1
  Add/1 -> C_m_T/1
  Selector2/1 -> C_m/3
  beta/1 -> C_m/2

== system DBX_model_all/Aeromodel/Aero model V1/Aerodynamics/Moment Coefficients/C_n_T ==
  note: Deflexiones efectivas:
      |
      | delta_ail_Asim
      | delta_rv_sim
      | delta_rv_Asim
  alpha : Inport
  beta : Inport  Port=2
  body_rates_adim : Inport  Port=3  PortDimensions=[3 1]
  defl_control : Inport  Port=4
  Add : Sum  Inputs=+++++
  C_n : Lookup_n-D  BreakpointsForDimension1=Alpha_unique_rad  BreakpointsForDimension2=Beta_unique_rad  Table=C_n  DiagnosticForOutOfRangeInput=Warning  RemoveProtectionInput=on  InternalRulePriority=Speed  RndMeth=Simplest  InputSameDT=on
  C_n_delta_a : Constant  Value=C_n_delta_a_Asim
  C_n_delta_rv : Constant  Value=C_n_delta_rv_Asim
  C_n_p : Constant  Value=C_n_p
  C_n_r : Constant  Value=C_n_r
  Divide{,1..3} (4 alike) : Product  Inputs=**
  Selector : Selector  InputPortWidth=3  Indices=3
  Selector1 : Selector  InputPortWidth=3  Indices=3
  Selector2 : Selector  InputPortWidth=3
  Selector3 : Selector  InputPortWidth=3
  C_n_T : Outport
  wires:
  alpha/1 -> C_n/1
  beta/1 -> C_n/2
  Add/1 -> C_n_T/1
  defl_control/1 -> Selector1/1, Selector2/1
  C_n_delta_a/1 -> Divide2/2
  Selector2/1 -> Divide2/1
  C_n_delta_rv/1 -> Divide1/2
  Selector1/1 -> Divide1/1
  C_n_r/1 -> Divide/2
  body_rates_adim/1 -> Selector3/1, Selector/1
  Selector3/1 -> Divide3/1
  C_n_p/1 -> Divide3/2
  Selector/1 -> Divide/1
  C_n/1 -> Add/1
  Divide/1 -> Add/2
  Divide3/1 -> Add/3
  Divide2/1 -> Add/4
  Divide1/1 -> Add/5

== system DBX_model_all/Aeromodel/Aero model V1/Aerodynamics/Wind-axes Velocities/Calculate alphadot ==
  note: Calculate alphadot
  note: W
  "[Udot Vdot Wdot]" : Inport
  "[U V W]" : Inport  Port=2
  Demux : Demux  Outputs=3
  Demux1 : Demux  Outputs=3
  Math Function : Math  Operator=square  SaturateOnIntegerOverflow=on
  Math Function1 : Math  Operator=square  SaturateOnIntegerOverflow=on
  Product : Product  RndMeth=Zero
  Product1 : Product  RndMeth=Zero
  Product2 : Product  Inputs=*/  RndMeth=Zero
  Sum : Sum  Inputs=-|+
  Sum1 : Sum  Inputs=+|+
  Terminator : Terminator
  Terminator1 : Terminator
  alphadot : Outport
  wires:
  Product2/1 -> alphadot/1  "alphadot"
  "[Udot Vdot Wdot]"/1 -> Demux/1
  "[U V W]"/1 -> Demux1/1
  Demux1/2 -> Terminator1/1
  Sum/1 -> Product2/1
  Product/1 -> Sum/2  "U Wdot"
  Product1/1 -> Sum/1  "W Udot"
  Sum1/1 -> Product2/2  "U^2 + W^2"
  Math Function1/1 -> Sum1/2
  Math Function/1 -> Sum1/1
  Demux1/3 -> Math Function1/1, Product1/2
  Demux1/1 -> Math Function/1, Product/2  "U"
  Demux/2 -> Terminator/1
  Demux/3 -> Product/1  "Wdot"
  Demux/1 -> Product1/1  "Udot"

== system DBX_model_all/Aeromodel/Aero model V2/Aerodynamics/Force Coefficients/C_X_T ==
  note: Deflexiones del modelo Aero:
      |
      | delta_ail
      | delta_elev
      | delta_rudder
  alpha : Inport
  beta : Inport  Port=2
  body_rates_adim : Inport  Port=3  PortDimensions=[3 1]
  defl_control : Inport  Port=4
  Abs : Abs
  Add : Sum  Inputs=+++
  Add1 : Sum  Inputs=-+|
  C_D_q : Constant  Value=DBX_aero.C_D_q
  C_Lift_q : Constant  Value=DBX_aero.C_Lift_q
  C_X : Lookup_n-D  BreakpointsForDimension1=DBX_aero.alpha_rad  BreakpointsForDimension2=DBX_aero.beta_rad  BreakpointsForDimension3=delta_elev_unique_rad  BeginIndexSearchUsingPreviousIndexResult=on  Table=DBX_aero.C_X  ExtrapMethod=Clip  DiagnosticForOutOfRangeInput=Warning  RemoveProtectionInput=on  InternalRulePriority=Speed  RndMeth=Simplest  InputSameDT=on
  C_X_delta_elev : Lookup_n-D  BreakpointsForDimension1=DBX_aero.alpha_rad  BreakpointsForDimension2=DBX_aero.delta_elev_rad  BreakpointsForDimension3=delta_elev_unique_rad  BeginIndexSearchUsingPreviousIndexResult=on  Table=DBX_aero.C_X_delta_elev  ExtrapMethod=Clip  DiagnosticForOutOfRangeInput=Warning  RemoveProtectionInput=on  InternalRulePriority=Speed  RndMeth=Simplest  InputSameDT=on
  Divide : Product  Inputs=**
  Divide1 : Product  Inputs=**
  Divide2 : Product  Inputs=**
  Selector : Selector  InputPortWidth=3  Indices=2
  Selector1 : Selector  InputPortWidth=3  Indices=2
  cos : Trigonometry  Operator=cos
  sin : Trigonometry
  C_X_T : Outport
  wires:
  Divide2/1 -> Add1/1
  Divide1/1 -> Add1/2
  C_D_q/1 -> Divide2/2
  cos/1 -> Divide2/1
  C_Lift_q/1 -> Divide1/2
  sin/1 -> Divide1/1
  defl_control/1 -> Selector1/1
  Add/1 -> C_X_T/1
  Divide/1 -> Add/3
  Selector/1 -> Divide/2
  body_rates_adim/1 -> Selector/1
  beta/1 -> Abs/1
  alpha/1 -> cos/1, C_X_delta_elev/1, sin/1, C_X/1
  Selector1/1 -> C_X_delta_elev/2
  C_X_delta_elev/1 -> Add/2
  Add1/1 -> Divide/1
  C_X/1 -> Add/1
  Abs/1 -> C_X/2

== system DBX_model_all/Aeromodel/Aero model V2/Aerodynamics/Force Coefficients/C_Y_T ==
  note: Deflexiones del modelo Aero:
      |
      | delta_ail
      | delta_elev
      | delta_rudder
  alpha : Inport
  beta : Inport  Port=2
  body_rates_adim : Inport  Port=3  PortDimensions=[3 1]
  defl_control : Inport  Port=4
  Abs : Abs
  Add : Sum  Inputs=++++
  C_Y : Lookup_n-D  BreakpointsForDimension1=DBX_aero.alpha_rad  BreakpointsForDimension2=DBX_aero.beta_rad  BreakpointsForDimension3=delta_elev_unique_rad  BeginIndexSearchUsingPreviousIndexResult=on  Table=DBX_aero.C_Y  ExtrapMethod=Clip  DiagnosticForOutOfRangeInput=Warning  RemoveProtectionInput=on  InternalRulePriority=Speed  RndMeth=Simplest  InputSameDT=on
  C_Y_delta_rudd : Constant  Value=DBX_aero.C_Y_delta_rud
  C_Y_p : Constant  Value=DBX_aero.C_Y_p
  C_Y_r : Constant  Value=DBX_aero.C_Y_r
  Divide : Product  Inputs=**
  Divide1 : Product  Inputs=**
  Divide2 : Product  Inputs=**
  Product : Product
  Selector : Selector  InputPortWidth=3  Indices=3
  Selector1 : Selector  InputPortWidth=3
  Selector2 : Selector  InputPortWidth=3  Indices=3
  Sign : Signum
  C_Y_T : Outport
  wires:
  Add/1 -> C_Y_T/1
  Divide/1 -> Add/2
  Divide1/1 -> Add/3
  Divide2/1 -> Add/4
  Selector2/1 -> Divide2/1
  C_Y_delta_rudd/1 -> Divide2/2
  defl_control/1 -> Selector2/1
  C_Y_p/1 -> Divide1/2
  Selector1/1 -> Divide1/1
  body_rates_adim/1 -> Selector/1, Selector1/1
  C_Y_r/1 -> Divide/2
  Selector/1 -> Divide/1
  beta/1 -> Sign/1, Abs/1
  alpha/1 -> C_Y/1
  Sign/1 -> Product/2
  C_Y/1 -> Product/1
  Product/1 -> Add/1
  Abs/1 -> C_Y/2

== system DBX_model_all/Aeromodel/Aero model V2/Aerodynamics/Force Coefficients/C_Z_T ==
  note: Deflexiones del modelo Aero:
      |
      | delta_ail
      | delta_elev
      | delta_rudder
  alpha : Inport
  beta : Inport  Port=2
  body_rates_adim : Inport  Port=3  PortDimensions=[3 1]
  defl_control : Inport  Port=4
  Abs : Abs
  Add : Sum  Inputs=+++
  Add2 : Sum  Inputs=--|
  C_D_q : Constant  Value=DBX_aero.C_D_q
  C_Lift_q : Constant  Value=DBX_aero.C_Lift_q
  C_Z : Lookup_n-D  BreakpointsForDimension1=DBX_aero.alpha_rad  BreakpointsForDimension2=DBX_aero.beta_rad  BreakpointsForDimension3=delta_elev_unique_rad  BeginIndexSearchUsingPreviousIndexResult=on  Table=DBX_aero.C_Z  ExtrapMethod=Clip  DiagnosticForOutOfRangeInput=Warning  RemoveProtectionInput=on  InternalRulePriority=Speed  RndMeth=Simplest  InputSameDT=on
  C_Z_delta_elev : Lookup_n-D  BreakpointsForDimension1=DBX_aero.alpha_rad  BreakpointsForDimension2=DBX_aero.delta_elev_rad  BreakpointsForDimension3=delta_elev_unique_rad  BeginIndexSearchUsingPreviousIndexResult=on  Table=DBX_aero.C_Z_delta_elev  ExtrapMethod=Clip  DiagnosticForOutOfRangeInput=Warning  RemoveProtectionInput=on  InternalRulePriority=Speed  RndMeth=Simplest  InputSameDT=on
  Divide : Product  Inputs=**
  Divide4 : Product  Inputs=**
  Divide5 : Product  Inputs=**
  Selector : Selector  InputPortWidth=3  Indices=2
  Selector1 : Selector  InputPortWidth=3  Indices=2
  cos1 : Trigonometry  Operator=cos
  sin1 : Trigonometry
  C_Z_T : Outport
  wires:
  Add2/1 -> Divide/1
  C_Z_delta_elev/1 -> Add/2
  Selector1/1 -> C_Z_delta_elev/2
  beta/1 -> Abs/1
  body_rates_adim/1 -> Selector/1
  Selector/1 -> Divide/2
  Divide/1 -> Add/3
  Add/1 -> C_Z_T/1
  defl_control/1 -> Selector1/1
  sin1/1 -> Divide5/1
  Divide5/1 -> Add2/1
  Divide4/1 -> Add2/2
  C_D_q/1 -> Divide5/2
  C_Lift_q/1 -> Divide4/2
  cos1/1 -> Divide4/1
  alpha/1 -> C_Z/1, C_Z_delta_elev/1, sin1/1, cos1/1
  C_Z/1 -> Add/1
  Abs/1 -> C_Z/2

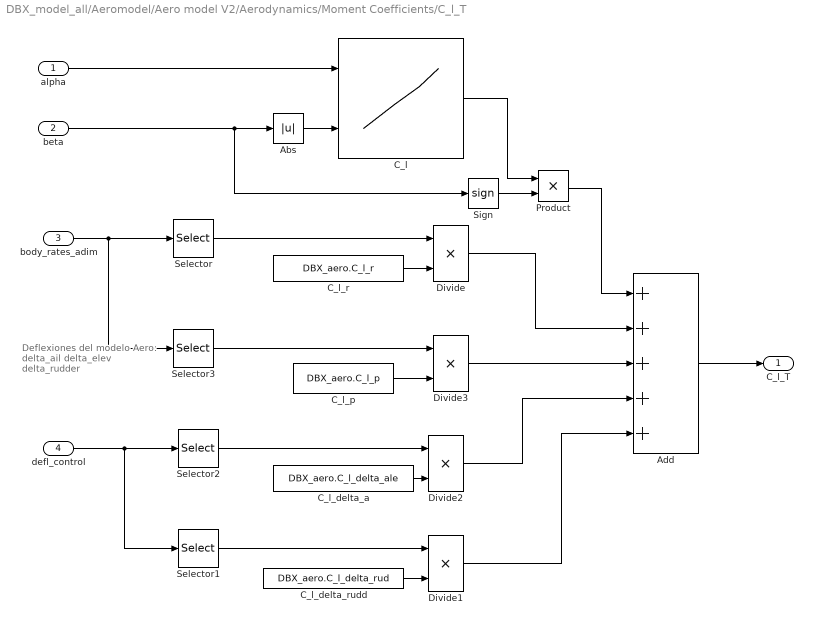
== system DBX_model_all/Aeromodel/Aero model V2/Aerodynamics/Moment Coefficients/C_l_T ==
  note: Deflexiones del modelo Aero:
      |
      | delta_ail
      | delta_elev
      | delta_rudder
  alpha : Inport
  beta : Inport  Port=2
  body_rates_adim : Inport  Port=3  PortDimensions=[3 1]
  defl_control : Inport  Port=4
  Abs : Abs
  Add : Sum  Inputs=+++++
  C_l : Lookup_n-D  BreakpointsForDimension1=DBX_aero.alpha_rad  BreakpointsForDimension2=DBX_aero.beta_rad  BreakpointsForDimension3=delta_elev_unique_rad  BeginIndexSearchUsingPreviousIndexResult=on  Table=DBX_aero.C_l  ExtrapMethod=Clip  DiagnosticForOutOfRangeInput=Warning  RemoveProtectionInput=on  InternalRulePriority=Speed  RndMeth=Simplest  InputSameDT=on
  C_l_delta_a : Constant  Value=DBX_aero.C_l_delta_ale
  C_l_delta_rudd : Constant  Value=DBX_aero.C_l_delta_rud
  C_l_p : Constant  Value=DBX_aero.C_l_p
  C_l_r : Constant  Value=DBX_aero.C_l_r
  Divide{,1..3} (4 alike) : Product  Inputs=**
  Product : Product
  Selector : Selector  InputPortWidth=3  Indices=3
  Selector1 : Selector  InputPortWidth=3  Indices=3
  Selector2 : Selector  InputPortWidth=3
  Selector3 : Selector  InputPortWidth=3
  Sign : Signum
  C_l_T : Outport
  wires:
  Divide1/1 -> Add/5
  Divide2/1 -> Add/4
  Divide3/1 -> Add/3
  Divide/1 -> Add/2
  Product/1 -> Add/1
  Selector/1 -> Divide/1
  C_l_p/1 -> Divide3/2
  Selector3/1 -> Divide3/1
  body_rates_adim/1 -> Selector/1, Selector3/1
  C_l_r/1 -> Divide/2
  Selector1/1 -> Divide1/1
  C_l_delta_rudd/1 -> Divide1/2
  Selector2/1 -> Divide2/1
  C_l_delta_a/1 -> Divide2/2
  defl_control/1 -> Selector2/1, Selector1/1
  Add/1 -> C_l_T/1
  beta/1 -> Sign/1, Abs/1
  alpha/1 -> C_l/1
  Abs/1 -> C_l/2
  Sign/1 -> Product/2
  C_l/1 -> Product/1

== system DBX_model_all/Aeromodel/Aero model V2/Aerodynamics/Moment Coefficients/C_m_T ==
  note: Deflexiones del modelo Aero:
      |
      | delta_ail
      | delta_elev
      | delta_rudder
  alpha : Inport
  beta : Inport  Port=2
  body_rates_adim : Inport  Port=3  PortDimensions=[3 1]
  defl_control : Inport  Port=4
  Abs : Abs
  Add : Sum  Inputs=+++|
  C_m : Lookup_n-D  BreakpointsForDimension1=DBX_aero.alpha_rad  BreakpointsForDimension2=DBX_aero.beta_rad  BreakpointsForDimension3=delta_elev_unique_rad  BeginIndexSearchUsingPreviousIndexResult=on  Table=DBX_aero.C_m  ExtrapMethod=Clip  DiagnosticForOutOfRangeInput=Warning  RemoveProtectionInput=on  InternalRulePriority=Speed  RndMeth=Simplest  InputSameDT=on
  C_m_delta_elev : Lookup_n-D  BreakpointsForDimension1=DBX_aero.alpha_rad  BreakpointsForDimension2=DBX_aero.delta_elev_rad  BreakpointsForDimension3=delta_elev_unique_rad  BeginIndexSearchUsingPreviousIndexResult=on  Table=DBX_aero.C_m_delta_elev  ExtrapMethod=Clip  DiagnosticForOutOfRangeInput=Warning  RemoveProtectionInput=on  InternalRulePriority=Speed  RndMeth=Simplest  InputSameDT=on
  C_m_q : Constant  Value=DBX_aero.C_m_q
  Divide : Product  Inputs=**
  Selector : Selector  InputPortWidth=3  Indices=2
  Selector2 : Selector  InputPortWidth=3  Indices=2
  C_m_T : Outport
  wires:
  Add/1 -> C_m_T/1
  C_m/1 -> Add/1
  Divide/1 -> Add/3
  defl_control/1 -> Selector2/1
  body_rates_adim/1 -> Selector/1
  C_m_q/1 -> Divide/2
  Selector/1 -> Divide/1
  beta/1 -> Abs/1
  alpha/1 -> C_m_delta_elev/1, C_m/1
  Abs/1 -> C_m/2
  Selector2/1 -> C_m_delta_elev/2
  C_m_delta_elev/1 -> Add/2

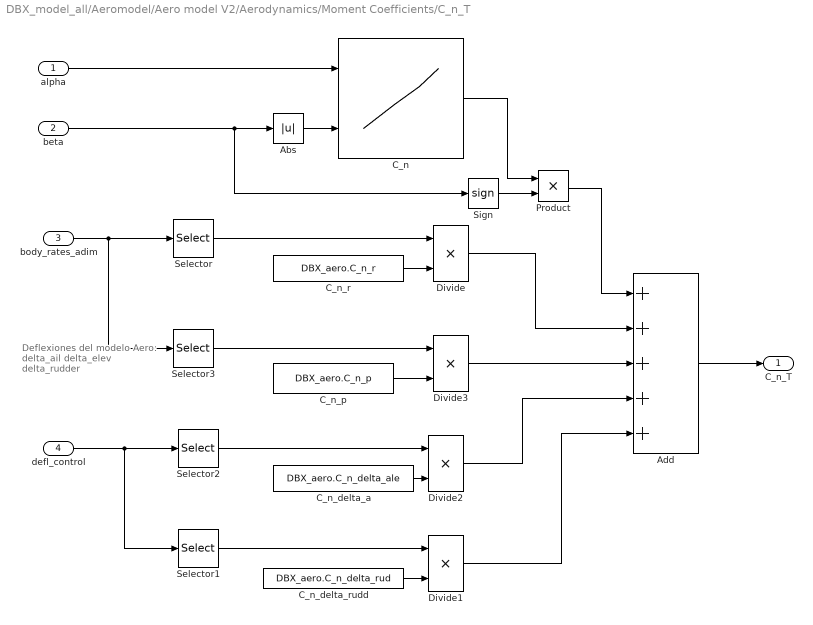
== system DBX_model_all/Aeromodel/Aero model V2/Aerodynamics/Moment Coefficients/C_n_T ==
  note: Deflexiones del modelo Aero:
      |
      | delta_ail
      | delta_elev
      | delta_rudder
  alpha : Inport
  beta : Inport  Port=2
  body_rates_adim : Inport  Port=3  PortDimensions=[3 1]
  defl_control : Inport  Port=4
  Abs : Abs
  Add : Sum  Inputs=+++++
  C_n : Lookup_n-D  BreakpointsForDimension1=DBX_aero.alpha_rad  BreakpointsForDimension2=DBX_aero.beta_rad  BreakpointsForDimension3=delta_elev_unique_rad  BeginIndexSearchUsingPreviousIndexResult=on  Table=DBX_aero.C_n  ExtrapMethod=Clip  DiagnosticForOutOfRangeInput=Warning  RemoveProtectionInput=on  InternalRulePriority=Speed  RndMeth=Simplest  InputSameDT=on
  C_n_delta_a : Constant  Value=DBX_aero.C_n_delta_ale
  C_n_delta_rudd : Constant  Value=DBX_aero.C_n_delta_rud
  C_n_p : Constant  Value=DBX_aero.C_n_p
  C_n_r : Constant  Value=DBX_aero.C_n_r
  Divide{,1..3} (4 alike) : Product  Inputs=**
  Product : Product
  Selector : Selector  InputPortWidth=3  Indices=3
  Selector1 : Selector  InputPortWidth=3  Indices=3
  Selector2 : Selector  InputPortWidth=3
  Selector3 : Selector  InputPortWidth=3
  Sign : Signum
  C_n_T : Outport
  wires:
  Divide1/1 -> Add/5
  Divide2/1 -> Add/4
  Divide3/1 -> Add/3
  Divide/1 -> Add/2
  Product/1 -> Add/1
  Selector/1 -> Divide/1
  C_n_p/1 -> Divide3/2
  Selector3/1 -> Divide3/1
  body_rates_adim/1 -> Selector/1, Selector3/1
  C_n_r/1 -> Divide/2
  Selector1/1 -> Divide1/1
  C_n_delta_rudd/1 -> Divide1/2
  Selector2/1 -> Divide2/1
  C_n_delta_a/1 -> Divide2/2
  defl_control/1 -> Selector2/1, Selector1/1
  Add/1 -> C_n_T/1
  beta/1 -> Sign/1, Abs/1
  alpha/1 -> C_n/1
  Abs/1 -> C_n/2
  Sign/1 -> Product/2
  C_n/1 -> Product/1

== system DBX_model_all/Aeromodel/Aero model V2/Aerodynamics/Wind-axes Velocities/Calculate alphadot ==
  note: W
  note: Calculate alphadot
  "[Udot Vdot Wdot]" : Inport
  "[U V W]" : Inport  Port=2
  Demux : Demux  Outputs=3
  Demux1 : Demux  Outputs=3
  Math Function : Math  Operator=square  SaturateOnIntegerOverflow=on
  Math Function1 : Math  Operator=square  SaturateOnIntegerOverflow=on
  Product : Product  RndMeth=Zero
  Product1 : Product  RndMeth=Zero
  Product2 : Product  Inputs=*/  RndMeth=Zero
  Sum : Sum  Inputs=-|+
  Sum1 : Sum  Inputs=+|+
  Terminator : Terminator
  Terminator1 : Terminator
  alphadot : Outport
  wires:
  Demux/1 -> Product1/1  "Udot"
  Demux/3 -> Product/1  "Wdot"
  Demux/2 -> Terminator/1
  Demux1/1 -> Product/2, Math Function/1  "U"
  Demux1/3 -> Product1/2, Math Function1/1
  Math Function/1 -> Sum1/1
  Math Function1/1 -> Sum1/2
  Sum1/1 -> Product2/2  "U^2 + W^2"
  Product1/1 -> Sum/1  "W Udot"
  Product/1 -> Sum/2  "U Wdot"
  Sum/1 -> Product2/1
  Demux1/2 -> Terminator1/1
  "[U V W]"/1 -> Demux1/1
  "[Udot Vdot Wdot]"/1 -> Demux/1
  Product2/1 -> alphadot/1  "alphadot"

== system DBX_model_all/Aeromodel/Aero model V2 parametric/Aerodynamics/Force Coefficients/C_X_T ==
  note: Deflexiones del modelo Aero:
      |
      | delta_ail
      | delta_elev
      | delta_rudder
  alpha : Inport
  beta : Inport  Port=2
  body_rates_adim : Inport  Port=3  PortDimensions=[3 1]
  defl_control : Inport  Port=4
  Add : Sum  Inputs=+++
  Add1 : Sum  Inputs=-+|
  C_D_q : Constant  Value=DBX_aero_param.C_D_q
  C_Lift_q : Constant  Value=DBX_aero_param.C_Lift_q
  C_X : Subsystem
  C_X_delta_elev : Subsystem
  Divide : Product  Inputs=**
  Divide1 : Product  Inputs=**
  Divide2 : Product  Inputs=**
  Selector : Selector  InputPortWidth=3  Indices=2
  Selector1 : Selector  InputPortWidth=3  Indices=2
  cos : Trigonometry  Operator=cos
  sin : Trigonometry
  C_X_T : Outport
  wires:
  Divide2/1 -> Add1/1
  Divide1/1 -> Add1/2
  C_D_q/1 -> Divide2/2
  cos/1 -> Divide2/1
  C_Lift_q/1 -> Divide1/2
  sin/1 -> Divide1/1
  defl_control/1 -> Selector1/1
  Add/1 -> C_X_T/1
  Divide/1 -> Add/3
  Selector/1 -> Divide/2
  body_rates_adim/1 -> Selector/1
  alpha/1 -> cos/1, C_X/1(x), sin/1, C_X_delta_elev/1(x)
  Selector1/1 -> C_X_delta_elev/2(y)
  C_X_delta_elev/1(C_X_delta_elev_out) -> Add/2
  Add1/1 -> Divide/1
  C_X/1(C_X_out) -> Add/1
  beta/1 -> C_X/2(y)

== system DBX_model_all/Aeromodel/Aero model V2 parametric/Aerodynamics/Force Coefficients/C_Y_T ==
  note: Deflexiones del modelo Aero:
      |
      | delta_ail
      | delta_elev
      | delta_rudder
  alpha : Inport
  beta : Inport  Port=2
  body_rates_adim : Inport  Port=3  PortDimensions=[3 1]
  defl_control : Inport  Port=4
  Add : Sum  Inputs=++++
  C_Y : Subsystem
  C_Y_delta_rudd : Constant  Value=DBX_aero_param.C_Y_delta_rud
  C_Y_p : Constant  Value=DBX_aero_param.C_Y_p
  C_Y_r : Constant  Value=DBX_aero_param.C_Y_r
  Divide : Product  Inputs=**
  Divide1 : Product  Inputs=**
  Divide2 : Product  Inputs=**
  Selector : Selector  InputPortWidth=3  Indices=3
  Selector1 : Selector  InputPortWidth=3
  Selector2 : Selector  InputPortWidth=3  Indices=3
  C_Y_T : Outport
  wires:
  Add/1 -> C_Y_T/1
  Divide/1 -> Add/2
  Divide1/1 -> Add/3
  Divide2/1 -> Add/4
  Selector2/1 -> Divide2/1
  C_Y_delta_rudd/1 -> Divide2/2
  defl_control/1 -> Selector2/1
  C_Y_p/1 -> Divide1/2
  Selector1/1 -> Divide1/1
  body_rates_adim/1 -> Selector/1, Selector1/1
  C_Y_r/1 -> Divide/2
  Selector/1 -> Divide/1
  beta/1 -> C_Y/2(y)
  alpha/1 -> C_Y/1(x)
  C_Y/1(C_Y_out) -> Add/1

== system DBX_model_all/Aeromodel/Aero model V2 parametric/Aerodynamics/Force Coefficients/C_Z_T ==
  note: Deflexiones del modelo Aero:
      |
      | delta_ail
      | delta_elev
      | delta_rudder
  alpha : Inport
  beta : Inport  Port=2
  body_rates_adim : Inport  Port=3  PortDimensions=[3 1]
  defl_control : Inport  Port=4
  Add : Sum  Inputs=+++
  Add2 : Sum  Inputs=--|
  C_D_q : Constant  Value=DBX_aero_param.C_D_q
  C_Lift_q : Constant  Value=DBX_aero_param.C_Lift_q
  C_Z : Subsystem
  C_Z_delta_elev : Subsystem
  Divide : Product  Inputs=**
  Divide4 : Product  Inputs=**
  Divide5 : Product  Inputs=**
  Selector : Selector  InputPortWidth=3  Indices=2
  Selector1 : Selector  InputPortWidth=3  Indices=2
  cos1 : Trigonometry  Operator=cos
  sin1 : Trigonometry
  C_Z_T : Outport
  wires:
  Add2/1 -> Divide/1
  C_Z_delta_elev/1(C_Z_delta_elev_out) -> Add/2
  Selector1/1 -> C_Z_delta_elev/2(y)
  beta/1 -> C_Z/2(y)
  body_rates_adim/1 -> Selector/1
  Selector/1 -> Divide/2
  Divide/1 -> Add/3
  Add/1 -> C_Z_T/1
  defl_control/1 -> Selector1/1
  sin1/1 -> Divide5/1
  Divide5/1 -> Add2/1
  Divide4/1 -> Add2/2
  C_D_q/1 -> Divide5/2
  C_Lift_q/1 -> Divide4/2
  cos1/1 -> Divide4/1
  alpha/1 -> C_Z/1(x), sin1/1, C_Z_delta_elev/1(x), cos1/1
  C_Z/1(C_Z_out) -> Add/1

== system DBX_model_all/Aeromodel/Aero model V2 parametric/Aerodynamics/Moment Coefficients/C_l_T ==
  note: Deflexiones del modelo Aero:
      |
      | delta_ail
      | delta_elev
      | delta_rudder
  alpha : Inport
  beta : Inport  Port=2
  body_rates_adim : Inport  Port=3  PortDimensions=[3 1]
  defl_control : Inport  Port=4
  Add : Sum  Inputs=+++++
  C_l : Subsystem
  C_l_delta_a : Constant  Value=DBX_aero_param.C_l_delta_ale
  C_l_delta_rudd : Constant  Value=DBX_aero_param.C_l_delta_rud
  C_l_p : Constant  Value=DBX_aero_param.C_l_p
  C_l_r : Constant  Value=DBX_aero_param.C_l_r
  Divide{,1..3} (4 alike) : Product  Inputs=**
  Selector : Selector  InputPortWidth=3  Indices=3
  Selector1 : Selector  InputPortWidth=3  Indices=3
  Selector2 : Selector  InputPortWidth=3
  Selector3 : Selector  InputPortWidth=3
  C_l_T : Outport
  wires:
  Divide1/1 -> Add/5
  Divide2/1 -> Add/4
  Divide3/1 -> Add/3
  Divide/1 -> Add/2
  Selector/1 -> Divide/1
  C_l_p/1 -> Divide3/2
  Selector3/1 -> Divide3/1
  body_rates_adim/1 -> Selector/1, Selector3/1
  C_l_r/1 -> Divide/2
  Selector1/1 -> Divide1/1
  C_l_delta_rudd/1 -> Divide1/2
  Selector2/1 -> Divide2/1
  C_l_delta_a/1 -> Divide2/2
  defl_control/1 -> Selector2/1, Selector1/1
  Add/1 -> C_l_T/1
  beta/1 -> C_l/2(y)
  alpha/1 -> C_l/1(x)
  C_l/1(C_l_out) -> Add/1

== system DBX_model_all/Aeromodel/Aero model V2 parametric/Aerodynamics/Moment Coefficients/C_m_T ==
  note: Deflexiones del modelo Aero:
      |
      | delta_ail
      | delta_elev
      | delta_rudder
  alpha : Inport
  beta : Inport  Port=2
  body_rates_adim : Inport  Port=3  PortDimensions=[3 1]
  defl_control : Inport  Port=4
  Add : Sum  Inputs=+++|
  C_m : Subsystem
  C_m_delta_elev : Subsystem
  C_m_q : Constant  Value=DBX_aero_param.C_m_q
  Divide : Product  Inputs=**
  Selector : Selector  InputPortWidth=3  Indices=2
  Selector2 : Selector  InputPortWidth=3  Indices=2
  C_m_T : Outport
  wires:
  Add/1 -> C_m_T/1
  C_m/1(C_m_out) -> Add/1
  Divide/1 -> Add/3
  defl_control/1 -> Selector2/1
  body_rates_adim/1 -> Selector/1
  C_m_q/1 -> Divide/2
  Selector/1 -> Divide/1
  beta/1 -> C_m/2(y)
  alpha/1 -> C_m_delta_elev/1(x), C_m/1(x)
  Selector2/1 -> C_m_delta_elev/2(y)
  C_m_delta_elev/1(C_m_delta_elev_out) -> Add/2
